simulink model "responce_to_Msig"  (R2020a)
settings: Solver=VariableStepAuto  StartTime=0.0  StopTime=20  RelTol=1e-3
undefined symbols (not defined in the file or in its folder): duration, effort, index, joint_name, left_front, left_rear, model_name, right_front, right_rear, robotracer
libraries: robotgazebolib x16, simulink x1
settings Model: Creator=under  LastModifiedBy=under

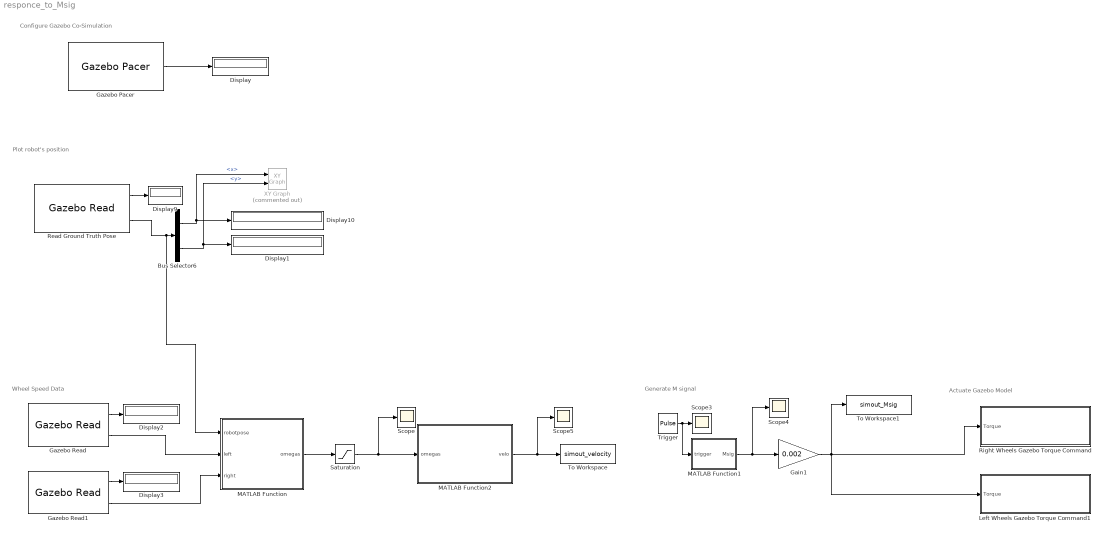
== system responce_to_Msig ==
  note: Configure Gazebo Co-Simulation
  note: Plot robot's position
  note: Generate M signal
  note: Wheel Speed Data
  note: Actuate Gazebo Model
  Bus Selector6 : BusSelector  OutputSignals=position.x,position.y
  Display{,1..3,9..10} (6 alike) : Display
  Gain1 : Gain  Gain=0.002
  Gazebo Pacer : robotgazebolib/Gazebo Pacer  ResetBehavior=Reset Gazebo simulation time and scene  SampleTime=0.001
      settings: SourceProductBaseCode=RO
  Gazebo Read : robotgazebolib/Gazebo Read  topicSource=From Gazebo  topic=/gazebo/ground_truth/world_pose/robotracer/left_front_wheel  messageType=gazebo_msgs/Pose  sampleTime=0.001
      settings: SourceProductBaseCode=RO
  Gazebo Read1 : robotgazebolib/Gazebo Read  topicSource=From Gazebo  topic=/gazebo/ground_truth/world_pose/robotracer/right_front_wheel  messageType=gazebo_msgs/Pose  sampleTime=0.001
      settings: SourceProductBaseCode=RO
  Left Wheels Gazebo Torque Command1 : Subsystem
  MATLAB Function : MATLAB Function  TreatAsAtomicUnit=on
  MATLAB Function1 : MATLAB Function  TreatAsAtomicUnit=on
  MATLAB Function2 : MATLAB Function  TreatAsAtomicUnit=on
  Read Ground Truth Pose : robotgazebolib/Gazebo Read  topicSource=From Gazebo  topic=/gazebo/ground_truth/world_pose/robotracer/chassis  messageType=gazebo_msgs/Pose  sampleTime=0.001
      settings: SourceProductBaseCode=RO
  Right Wheels Gazebo Torque Command : Subsystem
  Saturation : Saturate  UpperLimit=90  LowerLimit=-90
  Scope{,3..5} (4 alike) : Scope
  To Workspace : ToWorkspace  VariableName=simout_velocity  SaveFormat=Timeseries  SampleTime=-1
  To Workspace1 : ToWorkspace  VariableName=simout_Msig  SaveFormat=Timeseries  SampleTime=-1
  Trigger : DiscretePulseGenerator  PulseType=Time based  Period=0.1  PulseWidth=50
  XY Graph : simulink/Sinks/XY Graph  Commented=on  xmin=-1  xmax=1  ymin=-1  ymax=1  st=-1
  wires:
  Gazebo Pacer/1 -> Display/1
  Bus Selector6/1 -> XY Graph/1, Display10/1  "<x>"
  Bus Selector6/2 -> XY Graph/2, Display1/1  "<y>"
  MATLAB Function/1(omegas) -> Saturation/1
  Read Ground Truth Pose/2 -> MATLAB Function/1(robotpose), Bus Selector6/1
  Gazebo Read1/2 -> MATLAB Function/3(right)
  Gazebo Read/2 -> MATLAB Function/2(left)
  Gazebo Read1/1 -> Display3/1
  Gazebo Read/1 -> Display2/1
  Gain1/1 -> To Workspace1/1, Right Wheels Gazebo Torque Command/1(Torque), Left Wheels Gazebo Torque Command1/1(Torque)
  Read Ground Truth Pose/1 -> Display9/1
  Saturation/1 -> MATLAB Function2/1(omegas), Scope/1
  MATLAB Function1/1(Msig) -> Gain1/1, Scope4/1
  Trigger/1 -> MATLAB Function1/1(trigger), Scope3/1
  MATLAB Function2/1(velo) -> Scope5/1, To Workspace/1

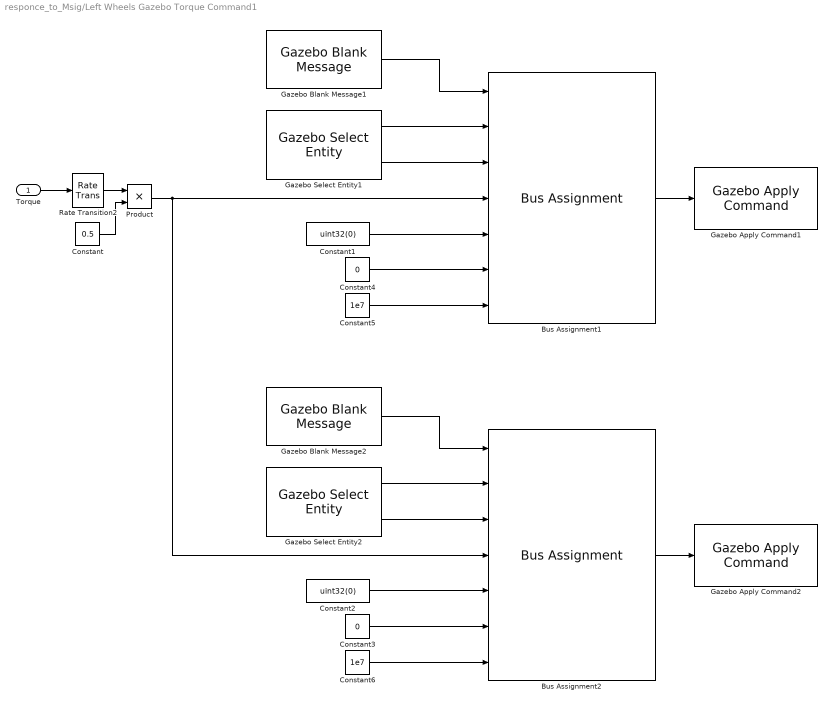
== system responce_to_Msig/Left Wheels Gazebo Torque Command1 ==
  Torque : Inport
  Bus Assignment1 : BusAssignment  AssignedSignals=model_name,joint_name,effort,index,duration.seconds,duration.nano_seconds
  Bus Assignment2 : BusAssignment  AssignedSignals=model_name,joint_name,effort,index,duration.seconds,duration.nano_seconds
  Constant : Constant  Value=0.5
  Constant1 : Constant  Value=uint32(0)
  Constant2 : Constant  Value=uint32(0)
  Constant3 : Constant  Value=0
  Constant4 : Constant  Value=0
  Constant5 : Constant  Value=1e7
  Constant6 : Constant  Value=1e7
  Gazebo Apply Command1 : robotgazebolib/Gazebo Apply Command  cmdType=ApplyJointTorque  sampleTime=0.01
      settings: SourceProductBaseCode=RO
  Gazebo Apply Command2 : robotgazebolib/Gazebo Apply Command  cmdType=ApplyJointTorque  sampleTime=0.01
      settings: SourceProductBaseCode=RO
  Gazebo Blank Message1 : robotgazebolib/Gazebo Blank Message  msgType=ApplyJointTorque  sampleTime=0.01  busName='Gazebo_SL_Bus_gazebo_msgs_ApplyJointTorque'
      settings: SourceProductBaseCode=RO
  Gazebo Blank Message2 : robotgazebolib/Gazebo Blank Message  msgType=ApplyJointTorque  sampleTime=0.01  busName='Gazebo_SL_Bus_gazebo_msgs_ApplyJointTorque'
      settings: SourceProductBaseCode=RO
  Gazebo Select Entity1 : robotgazebolib/Gazebo Select Entity  modelElemName=robotracer/left_front  outputArraySize=128  OutputLabel=Joint  SelectType=Joint
      settings: SourceProductBaseCode=RO
  Gazebo Select Entity2 : robotgazebolib/Gazebo Select Entity  modelElemName=robotracer/left_rear  outputArraySize=128  OutputLabel=Joint  SelectType=Joint
      settings: SourceProductBaseCode=RO
  Product : Product
  Rate Transition2 : RateTransition
  wires:
  Bus Assignment1/1 -> Gazebo Apply Command1/1
  Constant5/1 -> Bus Assignment1/7
  Gazebo Blank Message1/1 -> Bus Assignment1/1
  Gazebo Select Entity1/2 -> Bus Assignment1/3
  Gazebo Select Entity1/1 -> Bus Assignment1/2
  Constant4/1 -> Bus Assignment1/6
  Constant1/1 -> Bus Assignment1/5
  Gazebo Select Entity2/1 -> Bus Assignment2/2
  Constant6/1 -> Bus Assignment2/7
  Constant2/1 -> Bus Assignment2/5
  Constant3/1 -> Bus Assignment2/6
  Gazebo Select Entity2/2 -> Bus Assignment2/3
  Torque/1 -> Rate Transition2/1
  Gazebo Blank Message2/1 -> Bus Assignment2/1
  Bus Assignment2/1 -> Gazebo Apply Command2/1
  Constant/1 -> Product/2
  Rate Transition2/1 -> Product/1
  Product/1 -> Bus Assignment2/4, Bus Assignment1/4

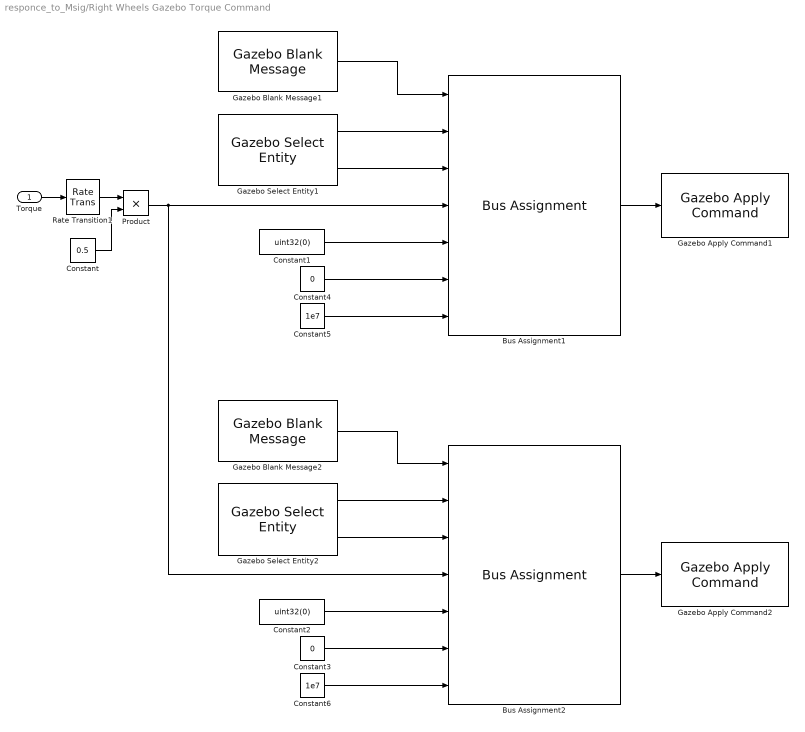
== system responce_to_Msig/Right Wheels Gazebo Torque Command ==
  Torque : Inport
  Bus Assignment1 : BusAssignment  AssignedSignals=model_name,joint_name,effort,index,duration.seconds,duration.nano_seconds
  Bus Assignment2 : BusAssignment  AssignedSignals=model_name,joint_name,effort,index,duration.seconds,duration.nano_seconds
  Constant : Constant  Value=0.5
  Constant1 : Constant  Value=uint32(0)
  Constant2 : Constant  Value=uint32(0)
  Constant3 : Constant  Value=0
  Constant4 : Constant  Value=0
  Constant5 : Constant  Value=1e7
  Constant6 : Constant  Value=1e7
  Gazebo Apply Command1 : robotgazebolib/Gazebo Apply Command  cmdType=ApplyJointTorque  sampleTime=0.001
      settings: SourceProductBaseCode=RO
  Gazebo Apply Command2 : robotgazebolib/Gazebo Apply Command  cmdType=ApplyJointTorque  sampleTime=0.001
      settings: SourceProductBaseCode=RO
  Gazebo Blank Message1 : robotgazebolib/Gazebo Blank Message  msgType=ApplyJointTorque  sampleTime=0.001  busName='Gazebo_SL_Bus_gazebo_msgs_ApplyJointTorque'
      settings: SourceProductBaseCode=RO
  Gazebo Blank Message2 : robotgazebolib/Gazebo Blank Message  msgType=ApplyJointTorque  sampleTime=0.001  busName='Gazebo_SL_Bus_gazebo_msgs_ApplyJointTorque'
      settings: SourceProductBaseCode=RO
  Gazebo Select Entity1 : robotgazebolib/Gazebo Select Entity  modelElemName=robotracer/right_front  outputArraySize=128  OutputLabel=Joint  SelectType=Joint
      settings: SourceProductBaseCode=RO
  Gazebo Select Entity2 : robotgazebolib/Gazebo Select Entity  modelElemName=robotracer/right_rear  outputArraySize=128  OutputLabel=Joint  SelectType=Joint
      settings: SourceProductBaseCode=RO
  Product : Product
  Rate Transition1 : RateTransition
  wires:
  Bus Assignment1/1 -> Gazebo Apply Command1/1
  Constant5/1 -> Bus Assignment1/7
  Gazebo Blank Message1/1 -> Bus Assignment1/1
  Gazebo Select Entity1/2 -> Bus Assignment1/3
  Gazebo Select Entity1/1 -> Bus Assignment1/2
  Constant4/1 -> Bus Assignment1/6
  Rate Transition1/1 -> Product/1
  Constant1/1 -> Bus Assignment1/5
  Gazebo Select Entity2/1 -> Bus Assignment2/2
  Constant6/1 -> Bus Assignment2/7
  Constant2/1 -> Bus Assignment2/5
  Constant3/1 -> Bus Assignment2/6
  Gazebo Select Entity2/2 -> Bus Assignment2/3
  Torque/1 -> Rate Transition1/1
  Gazebo Blank Message2/1 -> Bus Assignment2/1
  Bus Assignment2/1 -> Gazebo Apply Command2/1
  Constant/1 -> Product/2
  Product/1 -> Bus Assignment1/4, Bus Assignment2/4

== matlab function responce_to_Msig/MATLAB Function ==
  data: robotpose input; omegas output; left input; right input
function omegas = computeWheelVelocities(robotpose, left, right)
%computeWheelVelocities computes wheel velocity based on rate of change of
%the yaw angle of the wheel relative to its original mount on the robot
%body

persistent initAngles
if isempty(initAngles)
    initAngles = zeros(2, 1);
end
sampleTime = 0.001;

% compute rotation between wheel original mount on the robot body and world
% frame
robotRtom = quat2rotm([robotpose.orientation.w, robotpose.orientation.x, robotpose.orientation.y, robotpose.orientation.z]);
originalWheelMount = robotRtom * eul2rotm([pi/2 pi/2 0]);

% get rotation between wheel and the world frame
leftRtom = quat2rotm([left.orientation.w, left.orientation.x, left.orientation.y, left.orientation.z]);
rightRtom = quat2rotm([right.orientation.w, right.orientation.x, right.orientation.y, right.orientation.z]);

% compute relative rotation between wheel and its original mount
leftRotation = rotm2eul(originalWheelMount' * leftRtom);
rightRotation = rotm2eul(originalWheelMount' * rightRtom);

% compute angluar velocity using the angle difference between the current
% angle pose and the the angle pose in last time step
angles = [leftRotation(1); rightRotation(1)];
omegas = angdiff(initAngles, angles) / sampleTime;
if omegas(1, 1) < -1000
    omegas(1, 1) = 0;
end
if omegas(2, 1) < -1000
    omegas(2, 1) = 0;
end
initAngles = angles;

== matlab function responce_to_Msig/MATLAB Function1 ==
  data: trigger input; Msig output
function Msig = outputMsig(trigger)
    persistent signal
    persistent signal_size
    persistent pre_trigger
    persistent cnt
    persistent pre_Msig
    
    signal = [-1,-1,-1,-1,-1,1,-1,-1,-1,1,-1,-1,-1,1,1,-1,-1,1,-1,-1,-1,1,1,1,-1,1,-1,1,-1,1,1,-1,1,1,-1,-1,-1,1,1,1,-1,-1,-1,1,-1,-1,1,-1,1,-1,1,-1,-1,-1,1,1,-1,1,1,-1,-1,1,1,1,1,1,-1,-1,1,1,1,1,-1,-1,-1,1,-1,1,1,-1,1,1,1,-1,-1,1,-1,1,-1,-1,1,-1,-1,-1,-1,-1,1,-1,-1,1,1,-1,-1,1,1,1,-1,1,-1,-1,-1,1,1,1,1,1,-1,1,1,1,1,-1,-1,-1,-1,-1,1,1,1,1,1,1,1,1,1,-1,-1,-1,-1,1,1,1,1,-1,1,1,1,-1,-1,-1,-1,1,-1,1,1,-1,-1,1,1,-1,1,1,-1,1,1,1,1,-1,1,-1,-1,-1,-1,1,1,1,-1,-1,1,1,-1,-1,-1,-1,1,-1,-1,1,-1,-1,-1,1,-1,1,-1,1,1,1,-1,1];
    signal_size = length(signal, 1);
    
    if isempty(cnt)
        cnt = 1;
        pre_trigger = 0;
        pre_Msig = 0;
    end
        
    if pre_trigger == 0 && trigger == 1
        Msig = signal(cnt);
        cnt = cnt + 1;
        pre_Msig = Msig;
        disp(cnt);
    else 
        Msig = pre_Msig;
    end
    
    
    if cnt >= signal_size
        cnt = signal_size;
    end
    
    pre_trigger = trigger;

== matlab function responce_to_Msig/MATLAB Function2 ==
  data: omegas input; velo output
function velo = omegas2velocity(omegas)
    wheel_radius = 0.010; %[m]
    m_per_omega = 2 * pi * wheel_radius;
    
    velo = mean(omegas, 'all') * m_per_omega;
